simulink model "damping_measurement"  (R2015b)
settings: Solver=ode1  StartTime=0.0  StopTime=20  FixedStep=0.001  RelTol=1e-3
undefined symbols (not defined in the file): Serial_Port, Standard_Devices
libraries: rtwinlib x1
settings Model: Creator=dave  LastModifiedBy=dave

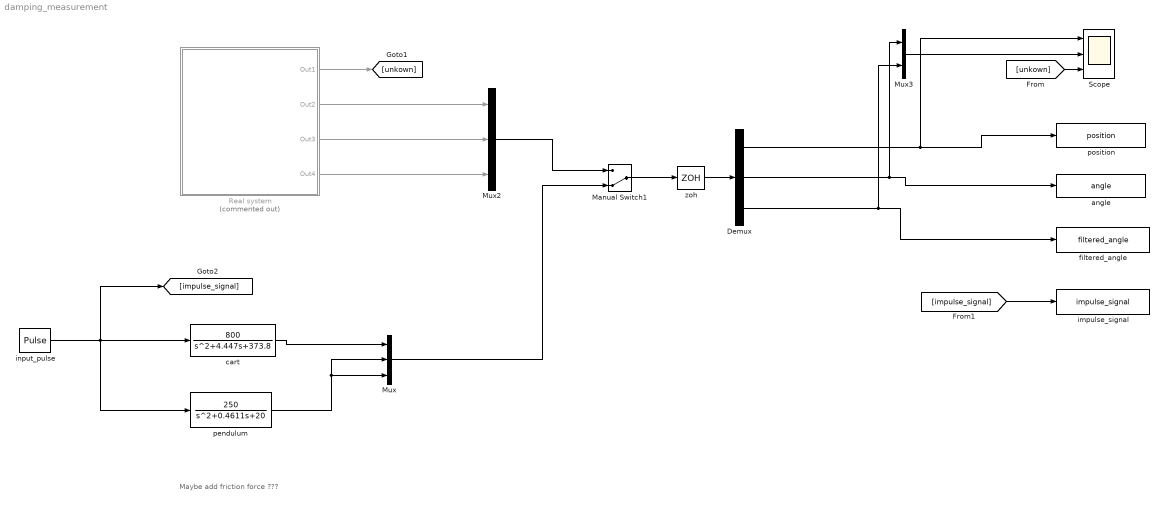
== system damping_measurement ==
  note: Maybe add friction force ???
  Demux : Demux  Outputs=3
  Manual Switch1 : ManualSwitch  CurrentSetting=0
  Mux : Mux  Inputs=3
  Mux2 : Mux  Inputs=3
  Mux3 : Mux  Inputs=2
  Real system : Subsystem  Commented=on
  Scope : Scope  NumInputPorts=3
  angle : ToWorkspace  VariableName=angle  SaveFormat=Timeseries  SampleTime=-1
  cart : TransferFcn  Numerator=[800]  Denominator=[1 4.447 373.8]
  filtered_angle : ToWorkspace  VariableName=filtered_angle  SaveFormat=Timeseries  SampleTime=-1
  impulse_signal : ToWorkspace  VariableName=impulse_signal  SaveFormat=Timeseries  SampleTime=-1
  input_pulse : DiscretePulseGenerator  PulseType=Time based  Amplitude=1000  Period=100  PulseWidth=0.001
  pendulum : TransferFcn  Numerator=[250]  Denominator=[1 0.4611 20]
  position : ToWorkspace  VariableName=position  SaveFormat=Timeseries  SampleTime=-1
  zoh : ZeroOrderHold  SampleTime=0.001
  wires:
  Real system/2(Out2) -> Mux2/1
  Real system/3(Out3) -> Mux2/2
  Real system/4(Out4) -> Mux2/3
  Mux2/1 -> Manual Switch1/1
  Manual Switch1/1 -> zoh/1
  Mux/1 -> Manual Switch1/2
  zoh/1 -> Demux/1
  Demux/2 -> Mux3/1, angle/1
  Demux/1 -> position/1, Scope/1
  Mux3/1 -> Scope/2
  Demux/3 -> Mux3/2, filtered_angle/1
  Real system/1(Out1) -> [unkown]
  [unkown] -> Scope/3
  cart/1 -> Mux/1
  pendulum/1 -> Mux/3, Mux/2
  [impulse_signal] -> impulse_signal/1
  input_pulse/1 -> pendulum/1, cart/1, [impulse_signal]

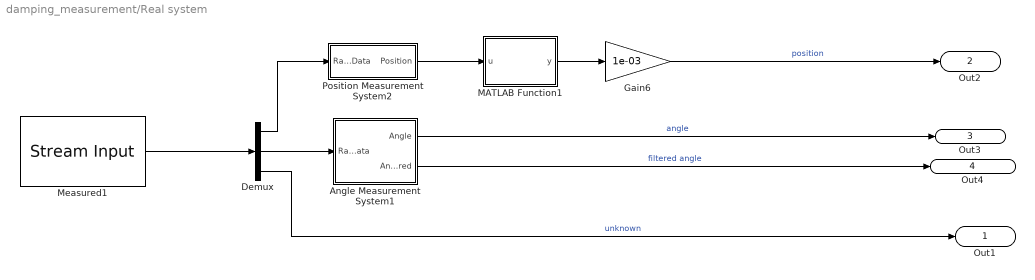
== system damping_measurement/Real system ==
  Angle Measurement System1 : Subsystem
  Demux : Demux  Outputs=3
  Gain6 : Gain  Gain=1e-03
  MATLAB Function1 : MATLAB Function  TreatAsAtomicUnit=on
  Measured1 : rtwinlib/Stream Input  SampleTime=0.001  MaxMissedTicks=inf  ShowMissedTicks=off  YieldWhenWaiting=off  DrvName=Standard_Devices/Serial_Port  DrvAddress=1  DrvOptions=[115200 8 0 0 0 0 0 1]  DataTypes='3*double'  FormatString='%f%f%f'  Terminator={'\r\n'}  ShowReady=off  ShowError=off
      settings: AttributesFormatString=Standard Devices\nSerial Port [1h]
  Position Measurement System2 : Subsystem
  Out1 : Outport
  Out2 : Outport  Port=2
  Out3 : Outport  Port=3
  Out4 : Outport  Port=4
  wires:
  Gain6/1 -> Out2/1  "position"
  Measured1/1 -> Demux/1
  Angle Measurement System1/2(Angle Filtered) -> Out4/1  "filtered angle"
  Angle Measurement System1/1(Angle) -> Out3/1  "angle"
  MATLAB Function1/1(y) -> Gain6/1
  Demux/2 -> Angle Measurement System1/1(RawData)
  Demux/3 -> Out1/1  "unknown"
  Position Measurement System2/1(Position) -> MATLAB Function1/1(u)
  Demux/1 -> Position Measurement System2/1(Raw Data)

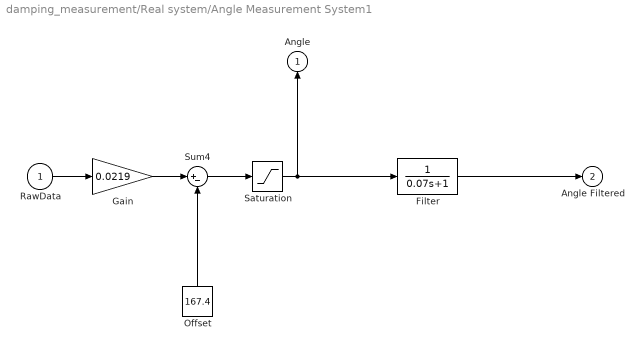
== system damping_measurement/Real system/Angle Measurement System1 ==
  RawData : Inport
  Filter : TransferFcn  Denominator=[0.07 1]
  Gain : Gain  Gain=0.0219
  Offset : Constant  Value=167.4  SampleTime=-1
  Saturation : Saturate  UpperLimit=90  LowerLimit=-90
  Sum4 : Sum  Inputs=|+-
  Angle : Outport
  Angle Filtered : Outport  Port=2
  wires:
  RawData/1 -> Gain/1
  Sum4/1 -> Saturation/1
  Gain/1 -> Sum4/1
  Offset/1 -> Sum4/2
  Filter/1 -> Angle Filtered/1
  Saturation/1 -> Filter/1, Angle/1

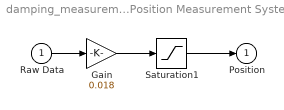
== system damping_measurement/Real system/Position Measurement System2 ==
  Raw Data : Inport
  Gain : Gain  Gain=0.018
  Saturation1 : Saturate  UpperLimit=1600  LowerLimit=0
  Position : Outport
  wires:
  Raw Data/1 -> Gain/1
  Saturation1/1 -> Position/1
  Gain/1 -> Saturation1/1

== matlab function damping_measurement/Real system/MATLAB Function1 ==
  data: u input; y output
function y = fcn(u)
%#codegen
if(0 <= u) && (u <= 600)
    y = u;
else
    y = u - 1179.576;
end
